simulink model "LidarMapSim128SeeWall"  (R2015b)
settings: Solver=ode3  StartTime=0.0  StopTime=inf  FixedStep=0.5  RelTol=1e-3
values from neighbouring files (symbols this model uses):
  REFMAP = [0 0 0 0 0 0 0 0 0 0 0 0 ... (65536 elements, 256x256)]    [Frontier256.mat]    (also in ParameterSet.m = MAP)
undefined symbols (not defined in the file or in its folder): Data, Data_SL_Info, Header, Info
libraries: robotlib x4
settings Model: Creator=einar  LastModifiedBy=saucer
settings OptimizationCC: OptimizeModelRefInitCode=on  LifeSpan=Inf  MaxStackSize=64
settings HardwareCC: ProdBitPerPointer=32  ProdLargestAtomicFloat=None  ProdIntDivRoundTo=Undefined  ProdEndianess=Unspecified  ProdWordSize=32  ProdHWDeviceType=Generic->Unspecified (assume 32-bit Generic)
settings RTWCC: SystemTargetFile=ert.tlc  TemplateMakefile=ert_default_tmf  Description=Embedded Coder  Toolchain=Catkin  TargetLang=C++
settings CodeAppCC: IgnoreCustomStorageClasses=off
settings ERTTargetCC: SupportVariableSizeSignals=on

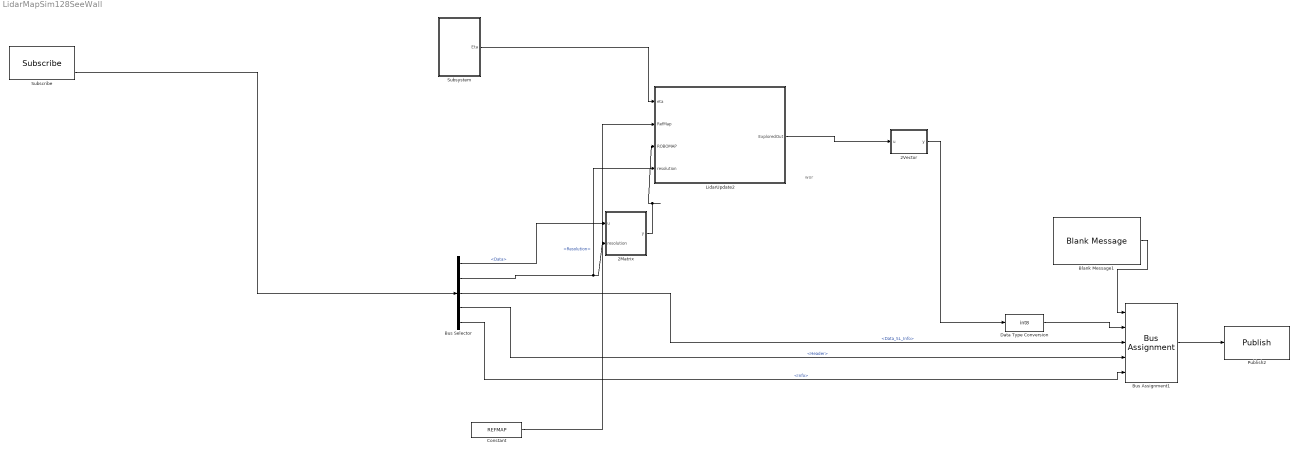
== system LidarMapSim128SeeWall ==
  note: wor
  2Matrix : MATLAB Function  TreatAsAtomicUnit=on
  2Vector : MATLAB Function  TreatAsAtomicUnit=on
  Blank Message1 : robotlib/Blank Message  SourceLibraryInfo=This block requires Robotics System Toolbox  messageType=nav_msgs/OccupancyGrid  SampleTime=inf
  Bus Assignment1 : BusAssignment  AssignedSignals=Data,Data_SL_Info,Header,Info
  Bus Selector : BusSelector  OutputSignals=Data,Info.Resolution,Data_SL_Info,Header,Info
  Constant : Constant  Value=REFMAP
  Data Type Conversion : DataTypeConversion  OutDataTypeStr=int8
  LidarUpdate2 : MATLAB Function  TreatAsAtomicUnit=on
  Publish2 : robotlib/Publish  SourceLibraryInfo=This block requires Robotics System Toolbox  topicSource=Specify your own  topic=/map  messageType=nav_msgs/OccupancyGrid  messageQueueLength=1
  Subscribe : robotlib/Subscribe  SourceLibraryInfo=This block requires Robotics System Toolbox  topicSource=Select from ROS network  topic=/map  messageType=nav_msgs/OccupancyGrid  sampleTime=0.5  messageQueueLength=1
  Subsystem : Subsystem
  wires:
  Bus Assignment1/1 -> Publish2/1
  Bus Selector/5 -> Bus Assignment1/5  "<Info>"
  Subsystem/1(Eta) -> LidarUpdate2/1(eta)
  Constant/1 -> LidarUpdate2/2(RefMap)
  Bus Selector/4 -> Bus Assignment1/4  "<Header>"
  Bus Selector/1 -> 2Matrix/1(u)  "<Data>"
  Subscribe/2 -> Bus Selector/1
  Bus Selector/2 -> LidarUpdate2/4(resolution), 2Matrix/2(resolution)  "<Resolution>"
  Blank Message1/1 -> Bus Assignment1/1
  2Matrix/1(y) -> LidarUpdate2/3(ROBOMAP)
  Bus Selector/3 -> Bus Assignment1/3  "<Data_SL_Info>"
  LidarUpdate2/1(ExploredOut) -> 2Vector/1(u)
  Data Type Conversion/1 -> Bus Assignment1/2
  2Vector/1(y) -> Data Type Conversion/1

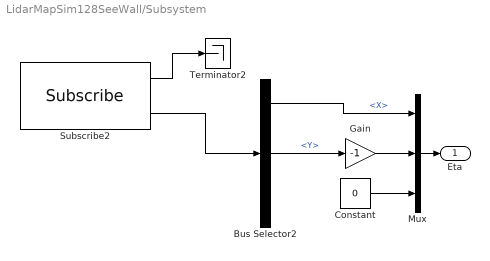
== system LidarMapSim128SeeWall/Subsystem ==
  Bus Selector2 : BusSelector  OutputSignals=X,Y,Z
  Constant : Constant  Value=0
  Gain : Gain  Gain=-1
  Mux : Mux  Inputs=3
  Subscribe2 : robotlib/Subscribe  SourceLibraryInfo=This block requires Robotics System Toolbox  topicSource=Specify your own  topic=/Eta  messageType=geometry_msgs/Vector3  sampleTime=-1  messageQueueLength=1
  Terminator2 : Terminator
  Eta : Outport
  wires:
  Bus Selector2/1 -> Mux/1  "<X>"
  Subscribe2/2 -> Bus Selector2/1
  Mux/1 -> Eta/1
  Subscribe2/1 -> Terminator2/1
  Bus Selector2/2 -> Gain/1  "<Y>"
  Constant/1 -> Mux/3
  Gain/1 -> Mux/2

== matlab function LidarMapSim128SeeWall/2Matrix ==
  data: u input; y output; resolution input
function y  = fcn(u,resolution)
K=sqrt(size(u,1));
%length(u)^0.5;
MAP=zeros(K,K);
for i=1:K;
    MAP(i,1:K)=u((i-1)*K+1:i*K);
end
y = (MAP);

== matlab function LidarMapSim128SeeWall/2Vector ==
  data: u input; y output
function y = fcn(u)
L=length(u);
y=zeros(L^2,1);
for i=1:L
y((i-1)*L+1:i*L)=u(i,:);
end

end

== matlab function LidarMapSim128SeeWall/LidarUpdate2 ==
  data: eta input; ExploredOut output; RefMap input; ROBOMAP input; resolution input
function ExploredOut=UpdateUserMap3(eta,RefMap,ROBOMAP,resolution)
[Height Width]=size(ROBOMAP);

MID=Height*resolution/2;
RobotPositionY=round((eta(1)+MID)/resolution);
RobotPositionX=round((eta(2)+MID)/resolution);

MAP=RefMap;
%ROBOMAP(RobotPositionX,RobotPositionY)=1;
for Degangle=0:1:360
    Radangle=Degangle*pi/180;
for r=0:0.5:6.5/resolution;
    XPOS=(RobotPositionX+round(r*cos(Radangle)));
    YPOS=RobotPositionY+round(r*sin(Radangle));
     if ( (XPOS>0) && (XPOS<1+size(ROBOMAP,2)) && (YPOS>0) &&(YPOS<1+size(ROBOMAP,1)) )
         if MAP(XPOS,YPOS)==0
     ROBOMAP(XPOS,YPOS)=0;
         end
 if MAP(XPOS,YPOS)==2
        ROBOMAP(XPOS,YPOS)=100;
        rEnd=r;
        break
        for r=0:0.5:rEnd-1;
    XPOS=(RobotPositionX+round(r*cos(Radangle)));
    YPOS=RobotPositionY+round(r*sin(Radangle));
        if MAP(XPOS,YPOS)==0
     ROBOMAP(XPOS,YPOS)=0;
     if ROBOMAP(XPOS,YPOS)==-1
         ROBOMAP(XPOS,YPOS)=0;
     end 
 end
        end
 break
 end
     end

end
end
ExploredOut=ROBOMAP;
end
